simulink model "modeloPlantaFenomenologico"  (R2014a)
settings: Solver=ode45  StartTime=0.0  StopTime=10.0  RelTol=1e-3
settings Model: Creator=Lab Automática  LastModifiedBy=Lab Automática

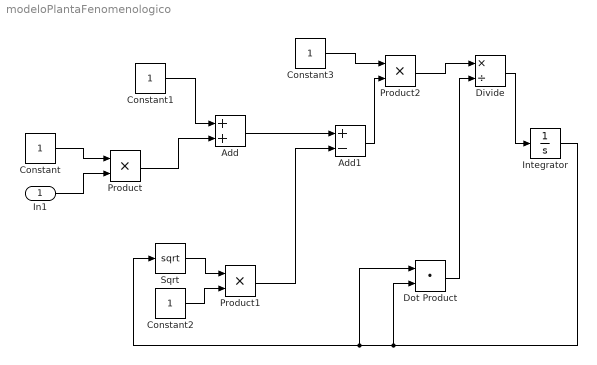
== system modeloPlantaFenomenologico ==
  In1 : Inport
  Add : Sum
  Add1 : Sum  Inputs=+-
  Constant{,1..3} (4 alike) : Constant
  Divide : Product  Inputs=*/
  Dot Product : DotProduct  InputSameDT=on  OutDataTypeStr=Inherit: Inherit via internal rule
  Integrator : Integrator
  Product : Product
  Product1 : Product
  Product2 : Product
  Sqrt : Sqrt  SaturateOnIntegerOverflow=on
  wires:
  In1/1 -> Product/2
  Constant/1 -> Product/1
  Product/1 -> Add/2
  Constant1/1 -> Add/1
  Constant2/1 -> Product1/2
  Sqrt/1 -> Product1/1
  Product1/1 -> Add1/2
  Add/1 -> Add1/1
  Integrator/1 -> Dot Product/2, Dot Product/1, Sqrt/1
  Add1/1 -> Product2/2
  Constant3/1 -> Product2/1
  Product2/1 -> Divide/1
  Dot Product/1 -> Divide/2
  Divide/1 -> Integrator/1
